simulink model "SimplifierDemo"  (R2012a)
settings: Solver=ode45  SolverMode=SingleTasking  StartTime=0.0  StopTime=10.0  RelTol=1e-3
libraries: simulink x1
settings Model: CovMetricSettings=dwe  CovHtmlReporting=off  covSaveCumulativeToWorkspaceVar=off  CovSaveSingleToWorkspaceVar=off  CovExternalEMLEnable=on  Creator=GM  LastModifiedBy=GM
settings DataIOCC: SaveFormat=StructureWithTime  ReturnWorkspaceOutputs=off
settings OptimizationCC: LifeSpan=inf  SimCompilerOptimization=Off
settings DebuggingCC: UnderspecifiedInitializationDetection=Classic  MergeDetectMultiDrivingBlocksExec=none  FcnCallInpInsideContextMsg=Enable All
settings HardwareCC: ProdWordSize=32  ProdHWDeviceType=Specified
settings SFSimCC: SimUseLocalCustomCode=off
settings RTWCC: RTWUseLocalCustomCode=off  RTWCompilerOptimization=Off
settings GRTTargetCC: CodeReplacementLibrary=C99 (ISO)  CPPClassGenCompliant=off

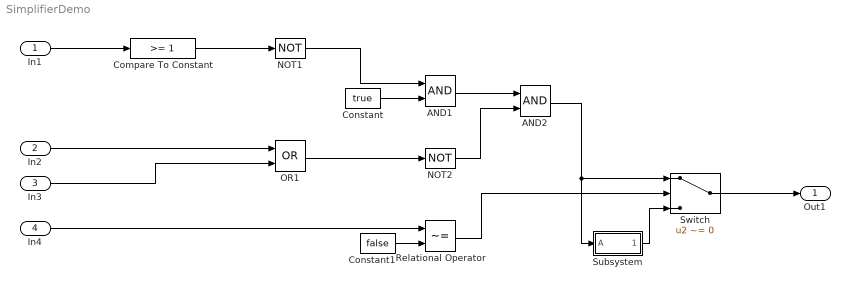
== system SimplifierDemo ==
  In1 : Inport
  In2 : Inport  Port=2
  In3 : Inport  Port=3
  In4 : Inport  Port=4
  AND1 : Logic  AllPortsSameDT=off  OutDataTypeStr=boolean
  AND2 : Logic  AllPortsSameDT=off  OutDataTypeStr=boolean
  Compare To Constant : simulink/Logic and Bit Operations/Compare To Constant  relop=>=  const=1  OutDataTypeStr=boolean
  Constant : Constant  Value=true
  Constant1 : Constant  Value=false
  NOT1 : Logic  Operator=NOT  AllPortsSameDT=off  OutDataTypeStr=boolean
  NOT2 : Logic  Operator=NOT  AllPortsSameDT=off  OutDataTypeStr=boolean
  OR1 : Logic  Operator=OR  AllPortsSameDT=off  OutDataTypeStr=boolean
  Relational Operator : RelationalOperator  Operator=~=  OutDataTypeStr=boolean
  Subsystem : Subsystem
  Switch : Switch  Criteria=u2 ~= 0
  Out1 : Outport
  wires:
  Subsystem/1(FALSE) -> Switch/3
  In2/1 -> OR1/1
  AND1/1 -> AND2/1
  NOT2/1 -> AND2/2
  NOT1/1 -> AND1/1
  In1/1 -> Compare To Constant/1
  AND2/1 -> Switch/1, Subsystem/1(A)
  Relational Operator/1 -> Switch/2
  Compare To Constant/1 -> NOT1/1
  In3/1 -> OR1/2
  OR1/1 -> NOT2/1
  Switch/1 -> Out1/1
  Constant/1 -> AND1/2
  Constant1/1 -> Relational Operator/2
  In4/1 -> Relational Operator/1

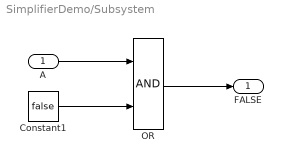
== system SimplifierDemo/Subsystem ==
  A : Inport
  Constant1 : Constant  Value=false
  OR : Logic  OutDataTypeStr=boolean
  FALSE : Outport
  wires:
  A/1 -> OR/1
  OR/1 -> FALSE/1
  Constant1/1 -> OR/2
